simulink model "Dracarys"  (R2024b)
settings: Solver=VariableStepAuto  StartTime=0.0  StopTime=10.0  RelTol=1e-3
undefined symbols (not defined in the file): D1, Delta
libraries: dspstat3 x8, spsThreePhaseVIMeasurementLib x6, spsThreePhaseTransformerTwoWindingsLib x5, spsThreePhaseBreakerLib x5, spsThreePhaseSourceLib x3, spsThreePhaseParallelRLCBranchLib x1, sps_lib x1
settings Model: Creator=ASUS  LastModifiedBy=ASUS

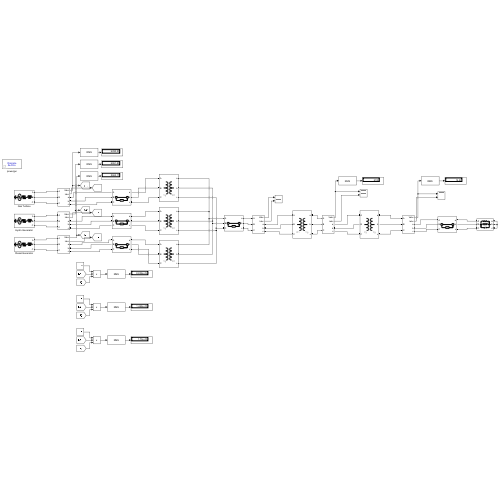
[thumbnail: Simulink's stored preview of the top-level diagram]
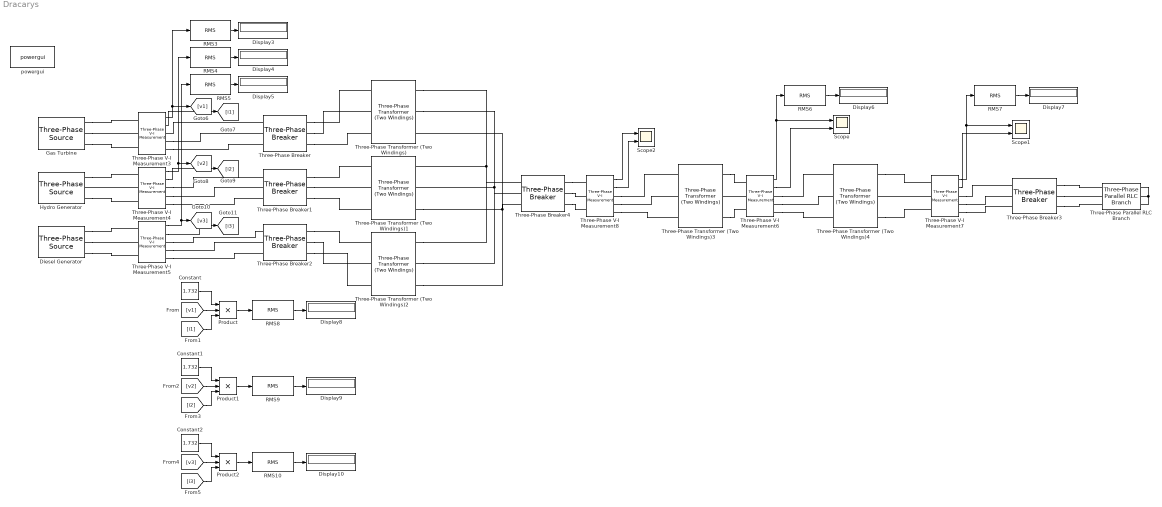
== system Dracarys ==
  Constant : Constant  Value=1.732
  Constant1 : Constant  Value=1.732
  Constant2 : Constant  Value=1.732
  Diesel Generator : spsThreePhaseSourceLib/Three-Phase Source  InternalConnection=Yg  VoltagePhases=off  Voltage=10e3  PhaseAngle=0  Voltage_phases=[25e3 25e3 25e3]/sqrt(3)  PhaseAngles_phases=[0 -120 +120]  Frequency=50  NonIdealSource=on  SpecifyImpedance=off  Resistance=0.6  Inductance=14e-3  ShortCircuitLevel=100e6  BaseVoltage=10e3  XRratio=7  BusType=PV  Pref=4e6  Qref=0  Prefabc=[10e3, 10e3, 10e3]  Qrefabc=[0, 0, 0]  Qmin=-2e6  Qmax=2e6
  Display{3..10} (8 alike) : Display
      Display3 settings: Format=bank
      Display4 settings: Format=bank
      Display5 settings: Format=bank
  Gas Turbine : spsThreePhaseSourceLib/Three-Phase Source  InternalConnection=Yg  VoltagePhases=off  Voltage=11e3  PhaseAngle=0  Voltage_phases=[25e3 25e3 25e3]/sqrt(3)  PhaseAngles_phases=[0 -120 +120]  Frequency=50  NonIdealSource=on  SpecifyImpedance=off  Resistance=0.8929  Inductance=16.58e-3  ShortCircuitLevel=100e6  BaseVoltage=11e3  XRratio=7  BusType=swing  Pref=10e3  Qref=0  Prefabc=[10e3, 10e3, 10e3]  Qrefabc=[0, 0, 0]  Qmin=-inf  Qmax=inf
  Hydro Generator : spsThreePhaseSourceLib/Three-Phase Source  InternalConnection=Yg  VoltagePhases=off  Voltage=12e3  PhaseAngle=0  Voltage_phases=[25e3 25e3 25e3]/sqrt(3)  PhaseAngles_phases=[0 -120 +120]  Frequency=50  NonIdealSource=on  SpecifyImpedance=off  Resistance=0.5  Inductance=12e-3  ShortCircuitLevel=100e6  BaseVoltage=12e3  XRratio=7  BusType=PV  Pref=2e6  Qref=0  Prefabc=[10e3, 10e3, 10e3]  Qrefabc=[0, 0, 0]  Qmin=-1e6  Qmax=1e6
  Product : Product  Inputs=3
  Product1 : Product  Inputs=3
  Product2 : Product  Inputs=3
  RMS{3..10} (8 alike) : dspstat3/RMS  run=off  directionMode=Each column  dimension=1  InputProcessing=Columns as channels (frame based)  reset_popup=None
  Scope : Scope  NumInputPorts=2
  Scope1 : Scope  NumInputPorts=2
  Scope2 : Scope  NumInputPorts=2
  Three-Phase Parallel RLC Branch : spsThreePhaseParallelRLCBranchLib/Three-Phase Parallel RLC Branch  LConnTagsString=A|B|C  RConnTagsString=A|B|C  BranchType=RLC  Resistance=1  Inductance=1e-3  Capacitance=1e-6  Measurements=None
  Three-Phase Transformer (Two Windings) : spsThreePhaseTransformerTwoWindingsLib/Three-Phase Transformer (Two Windings)  Winding1Connection=Yg  Winding2Connection=Delta (D1)  CoreType=Three single-phase transformers  SetSaturation=off  Hysteresis=off  DataFile='hysteresis'  SetInitialFlux=off  Measurements=None  UNITS=pu  NominalPower=[ 1.5e6 , 50 ]  Winding1=[ 11e3 , 0.01 , 0.08 ]  Winding2=[ 132e3 , 0.01 , 0.08 ]  Rm=500  Lm=30  L0=0.5  Saturation=[ 0,0 ; 0.0024,1.2 ; 1.0,1.52 ]  InitialFluxes=[ 0.8 , -0.8 , 0.7 ]  BreakLoop=off  DiscreteSolver=Trapezoidal iterative  DataType=off  TransfoNumber=1
  Three-Phase Transformer (Two Windings)1 : spsThreePhaseTransformerTwoWindingsLib/Three-Phase Transformer (Two Windings)  Winding1Connection=Yg  Winding2Connection=Delta (D1)  CoreType=Three single-phase transformers  SetSaturation=off  Hysteresis=off  DataFile='hysteresis'  SetInitialFlux=off  Measurements=None  UNITS=pu  NominalPower=[ 2.5e6 , 50 ]  Winding1=[ 12e3 , 0.01 , 0.08 ]  Winding2=[ 132e3 , 0.01 , 0.08 ]  Rm=500  Lm=30  L0=0.5  Saturation=[ 0,0 ; 0.0024,1.2 ; 1.0,1.52 ]  InitialFluxes=[ 0.8 , -0.8 , 0.7 ]  BreakLoop=off  DiscreteSolver=Trapezoidal iterative  DataType=off  TransfoNumber=1
  Three-Phase Transformer (Two Windings)2 : spsThreePhaseTransformerTwoWindingsLib/Three-Phase Transformer (Two Windings)  Winding1Connection=Yg  Winding2Connection=Delta (D1)  CoreType=Three single-phase transformers  SetSaturation=off  Hysteresis=off  DataFile='hysteresis'  SetInitialFlux=off  Measurements=None  UNITS=pu  NominalPower=[ 5e6 , 50 ]  Winding1=[ 10e3 , 0.01 , 0.08 ]  Winding2=[ 132e3 , 0.01 , 0.08 ]  Rm=500  Lm=30  L0=0.5  Saturation=[ 0,0 ; 0.0024,1.2 ; 1.0,1.52 ]  InitialFluxes=[ 0.8 , -0.8 , 0.7 ]  BreakLoop=off  DiscreteSolver=Trapezoidal iterative  DataType=off  TransfoNumber=1
  Three-Phase Transformer (Two Windings)3 : spsThreePhaseTransformerTwoWindingsLib/Three-Phase Transformer (Two Windings)  Winding1Connection=Delta (D1)  Winding2Connection=Yg  CoreType=Three single-phase transformers  SetSaturation=off  Hysteresis=off  DataFile='hysteresis'  SetInitialFlux=off  Measurements=None  UNITS=pu  NominalPower=[ 10e6 , 50 ]  Winding1=[ 132e3 , 0.01 , 0.08 ]  Winding2=[ 11e3 , 0.01 , 0.08 ]  Rm=500  Lm=30  L0=0.5  Saturation=[ 0,0 ; 0.0024,1.2 ; 1.0,1.52 ]  InitialFluxes=[ 0.8 , -0.8 , 0.7 ]  BreakLoop=off  DiscreteSolver=Trapezoidal iterative  DataType=off  TransfoNumber=1
  Three-Phase Transformer (Two Windings)4 : spsThreePhaseTransformerTwoWindingsLib/Three-Phase Transformer (Two Windings)  Winding1Connection=Yg  Winding2Connection=Yg  CoreType=Three single-phase transformers  SetSaturation=off  Hysteresis=off  DataFile='hysteresis'  SetInitialFlux=off  Measurements=None  UNITS=pu  NominalPower=[ 250e6 , 60 ]  Winding1=[ 735e3 , 0.002 , 0.08 ]  Winding2=[ 315e3 , 0.002 , 0.08 ]  Rm=500  Lm=500  L0=0.5  Saturation=[ 0,0 ; 0.0024,1.2 ; 1.0,1.52 ]  InitialFluxes=[ 0.8 , -0.8 , 0.7 ]  BreakLoop=off  DiscreteSolver=Trapezoidal iterative  DataType=off  TransfoNumber=1
  Three-Phase V-I Measurement{3..7} (5 alike) : spsThreePhaseVIMeasurementLib/Three-Phase V-I Measurement  VoltageMeasurement=phase-to-ground  SetLabelV=off  LabelV=Vabc  Vpu=off  VpuLL=off  CurrentMeasurement=yes  SetLabelI=off  LabelI=Iabc  Ipu=off  Pbase=100e6  Vbase=500e3  OutputType=Complex  PhasorSimulation=off  PSBequivalent=0
  Three-Phase V-I Measurement8 : spsThreePhaseVIMeasurementLib/Three-Phase V-I Measurement  VoltageMeasurement=phase-to-phase  SetLabelV=off  LabelV=Vabc  Vpu=off  VpuLL=off  CurrentMeasurement=yes  SetLabelI=off  LabelI=Iabc  Ipu=off  Pbase=100e6  Vbase=500e3  OutputType=Complex  PhasorSimulation=off  PSBequivalent=0
  Three-Phase Breaker{,1..4} (5 alike) : spsThreePhaseBreakerLib/Three-Phase Breaker  InitialState=closed  SwitchA=on  SwitchB=on  SwitchC=on  SwitchTimes="[1/60  5/60]"  External=off  BreakerResistance=0.01  SnubberResistance=1e6  SnubberCapacitance=inf  Measurements=None
  powergui : sps_lib/powergui  Priority=1  SimulationMode=Discrete  SampleTime=50e-6  frequency=60  Iterations=50  frequencyindice=0  Pbase=100e6  ErrMax=1e-4  UnitsV=kV  UnitsW=MW  buscounter=0  FunctionMessages=off  echomessages=off  EnableUseOfTLC=off  CurrentSourceSwitches=off  DisableSnubberDevices=off  DisableRonSwitches=off  DisableVfSwitches=off  DisplayEquations=off  AutomaticDiscreteSolvers=off  SolverType=Tustin/Backward Euler (TBE)  Interpol=off  ExternalGateDelay=off  methode=off  Ts=100  x0status=blocks  SPID=on  SwTol=0  HookPort=off  NonlinearTolerance=1e-4  nMaxIteration=100  ContinueOnMaxIteration=off  RestoreLinks=warning  ResistiveCurrentMeasurement=off  Frange=[0:2:500]  Ylog=off  Xlog=on  ShowGrid=off  save=off  variable=ZData  structure=0  ZoomFFT=off  StartTime=0.0  cycles=1  DisplayStyle=1  fundamental=60  FreqAxis=off  MaxFrequency=1000  frequencyindicesteady=1  RmsSteady=1  display=off
  wires:
  RMS3/1 -> Display3/1
  Three-Phase V-I Measurement3/1 -> [v1], RMS3/1
  RMS4/1 -> Display4/1
  Three-Phase V-I Measurement4/1 -> [v2], RMS4/1
  RMS5/1 -> Display5/1
  Three-Phase V-I Measurement5/1 -> [v3], RMS5/1
  RMS6/1 -> Display6/1
  Three-Phase V-I Measurement6/1 -> Scope/1, RMS6/1
  Three-Phase V-I Measurement6/2 -> Scope/2
  RMS7/1 -> Display7/1
  Three-Phase V-I Measurement7/1 -> Scope1/1, RMS7/1
  Three-Phase V-I Measurement7/2 -> Scope1/2
  Three-Phase V-I Measurement3/2 -> [i1]
  Three-Phase V-I Measurement4/2 -> [i2]
  Three-Phase V-I Measurement5/2 -> [i3]
  [v1] -> Product/2
  Constant/1 -> Product/1
  [i1] -> Product/3
  [i2] -> Product1/3
  [v2] -> Product1/2
  Constant1/1 -> Product1/1
  [i3] -> Product2/3
  [v3] -> Product2/2
  Constant2/1 -> Product2/1
  Product/1 -> RMS8/1
  RMS8/1 -> Display8/1
  RMS9/1 -> Display9/1
  Product1/1 -> RMS9/1
  Product2/1 -> RMS10/1
  RMS10/1 -> Display10/1
  Three-Phase V-I Measurement8/1 -> Scope2/1
  Three-Phase V-I Measurement8/2 -> Scope2/2
  connections:
  Three-Phase Breaker/RConn1 -- Three-Phase Transformer (Two Windings)/LConn1
  Three-Phase Breaker/RConn2 -- Three-Phase Transformer (Two Windings)/LConn2
  Three-Phase Breaker/RConn3 -- Three-Phase Transformer (Two Windings)/LConn3
  Three-Phase Breaker1/RConn1 -- Three-Phase Transformer (Two Windings)1/LConn1
  Three-Phase Breaker1/RConn2 -- Three-Phase Transformer (Two Windings)1/LConn2
  Three-Phase Breaker1/RConn3 -- Three-Phase Transformer (Two Windings)1/LConn3
  Three-Phase Breaker2/RConn1 -- Three-Phase Transformer (Two Windings)2/LConn1
  Three-Phase Breaker2/RConn2 -- Three-Phase Transformer (Two Windings)2/LConn2
  Three-Phase Breaker2/RConn3 -- Three-Phase Transformer (Two Windings)2/LConn3
  Three-Phase Parallel RLC Branch/RConn2 -- Three-Phase Parallel RLC Branch/RConn1 -- Three-Phase Parallel RLC Branch/RConn3
  Three-Phase Breaker3/RConn2 -- Three-Phase Parallel RLC Branch/LConn2
  Three-Phase Breaker3/RConn1 -- Three-Phase Parallel RLC Branch/LConn1
  Three-Phase Breaker3/RConn3 -- Three-Phase Parallel RLC Branch/LConn3
  Gas Turbine/RConn2 -- Three-Phase V-I Measurement3/LConn2
  Gas Turbine/RConn1 -- Three-Phase V-I Measurement3/LConn1
  Gas Turbine/RConn3 -- Three-Phase V-I Measurement3/LConn3
  Three-Phase V-I Measurement3/RConn2 -- Three-Phase Breaker/LConn2
  Three-Phase V-I Measurement3/RConn1 -- Three-Phase Breaker/LConn1
  Three-Phase V-I Measurement3/RConn3 -- Three-Phase Breaker/LConn3
  Three-Phase V-I Measurement4/LConn2 -- Hydro Generator/RConn2
  Hydro Generator/RConn1 -- Three-Phase V-I Measurement4/LConn1
  Hydro Generator/RConn3 -- Three-Phase V-I Measurement4/LConn3
  Three-Phase V-I Measurement4/RConn1 -- Three-Phase Breaker1/LConn1
  Three-Phase V-I Measurement4/RConn2 -- Three-Phase Breaker1/LConn2
  Three-Phase V-I Measurement4/RConn3 -- Three-Phase Breaker1/LConn3
  Diesel Generator/RConn2 -- Three-Phase V-I Measurement5/LConn2
  Diesel Generator/RConn1 -- Three-Phase V-I Measurement5/LConn1
  Diesel Generator/RConn3 -- Three-Phase V-I Measurement5/LConn3
  Three-Phase V-I Measurement5/RConn1 -- Three-Phase Breaker2/LConn1
  Three-Phase V-I Measurement5/RConn2 -- Three-Phase Breaker2/LConn2
  Three-Phase V-I Measurement5/RConn3 -- Three-Phase Breaker2/LConn3
  Three-Phase V-I Measurement6/LConn2 -- Three-Phase Transformer (Two Windings)3/RConn2
  Three-Phase Transformer (Two Windings)3/RConn1 -- Three-Phase V-I Measurement6/LConn1
  Three-Phase Transformer (Two Windings)3/RConn3 -- Three-Phase V-I Measurement6/LConn3
  Three-Phase V-I Measurement6/RConn1 -- Three-Phase Transformer (Two Windings)4/LConn1
  Three-Phase V-I Measurement6/RConn2 -- Three-Phase Transformer (Two Windings)4/LConn2
  Three-Phase V-I Measurement6/RConn3 -- Three-Phase Transformer (Two Windings)4/LConn3
  Three-Phase V-I Measurement7/LConn2 -- Three-Phase Transformer (Two Windings)4/RConn2
  Three-Phase V-I Measurement7/RConn2 -- Three-Phase Breaker3/LConn2
  Three-Phase V-I Measurement7/RConn1 -- Three-Phase Breaker3/LConn1
  Three-Phase V-I Measurement7/RConn3 -- Three-Phase Breaker3/LConn3
  Three-Phase Transformer (Two Windings)4/RConn1 -- Three-Phase V-I Measurement7/LConn1
  Three-Phase Transformer (Two Windings)4/RConn3 -- Three-Phase V-I Measurement7/LConn3
  Three-Phase V-I Measurement8/RConn1 -- Three-Phase Transformer (Two Windings)3/LConn1
  Three-Phase V-I Measurement8/RConn2 -- Three-Phase Transformer (Two Windings)3/LConn2
  Three-Phase V-I Measurement8/RConn3 -- Three-Phase Transformer (Two Windings)3/LConn3
  Three-Phase Transformer (Two Windings)/RConn1 -- Three-Phase Breaker4/LConn1 -- Three-Phase Transformer (Two Windings)2/RConn1 -- Three-Phase Transformer (Two Windings)1/RConn1
  Three-Phase Transformer (Two Windings)/RConn2 -- Three-Phase Breaker4/LConn2 -- Three-Phase Transformer (Two Windings)2/RConn2 -- Three-Phase Transformer (Two Windings)1/RConn2
  Three-Phase Transformer (Two Windings)1/RConn3 -- Three-Phase Breaker4/LConn3 -- Three-Phase Transformer (Two Windings)/RConn3 -- Three-Phase Transformer (Two Windings)2/RConn3
  Three-Phase Breaker4/RConn1 -- Three-Phase V-I Measurement8/LConn1
  Three-Phase Breaker4/RConn2 -- Three-Phase V-I Measurement8/LConn2
  Three-Phase Breaker4/RConn3 -- Three-Phase V-I Measurement8/LConn3
